simulink model "sf_frame_sync_controller"  (R2017b)
settings: Solver=FixedStepDiscrete  StartTime=0.0  StopTime=10.0  FixedStep=0.05  RelTol=1e-3  EnableMultiTasking=on
model workspace (MAT data in the model file):
  trainSig = [-0.707106781187+0.707106781187i; -0.707106781187+0.707106781187i; -0.707106781187+0.707106781187i; -0.707106781187+0.707106781187i; -0.707106781187-0.707106781187i; -0.707106781187-0.707106781187i; 0.707106781187-0.707106781187i; 0.707106781187-0.707106781187i; -0.707106781187-0.707106781187i; -0.707106781187+0.707106781187i; 0.707106781187-0.707106781187i; -0.707106781187-0.707106781187i; -0.707106781187+0.707106781187i; 0.707106781187-0.707106781187i; 0.707106781187-0.707106781187i; -0.707106781187-0.707106781187i; -0.707106781187-0.707106781187i; -0.707106781187-0.707106781187i; 0.707106781187+0.707106781187i; -0.707106781187+0.707106781187i; -0.707106781187+0.707106781187i; 0.707106781187+0.707106781187i; 0.707106781187-0.707106781187i; 0.707106781187+0.707106781187i; 0.707106781187+0.707106781187i; 0.707106781187+0.707106781187i; 0.707106781187+0.707106781187i; -0.707106781187+0.707106781187i; -0.707106781187+0.707106781187i; 0.707106781187-0.707106781187i; -0.707106781187+0.707106781187i; 0.707106781187+0.707106781187i; 0.707106781187-0.707106781187i; 0.707106781187-0.707106781187i; -0.707106781187+0.707106781187i; 0.707106781187+0.707106781187i; -0.707106781187+0.707106781187i; -0.707106781187+0.707106781187i; -0.707106781187-0.707106781187i; -0.707106781187+0.707106781187i; -0.707106781187-0.707106781187i; -0.707106781187-0.707106781187i; 0.707106781187+0.707106781187i; 0.707106781187+0.707106781187i; -0.707106781187+0.707106781187i; -0.707106781187+0.707106781187i; -0.707106781187+0.707106781187i; -0.707106781187-0.707106781187i; 0.707106781187+0.707106781187i; -0.707106781187+0.707106781187i; 0.707106781187-0.707106781187i; 0.707106781187+0.707106781187i; 0.707106781187-0.707106781187i; -0.707106781187-0.707106781187i; -0.707106781187+0.707106781187i; -0.707106781187-0.707106781187i; 0.707106781187+0.707106781187i; -0.707106781187+0.707106781187i; 0.707106781187-0.707106781187i; -0.707106781187-0.707106781187i; -0.707106781187-0.707106781187i; 0.707106781187+0.707106781187i; -0.707106781187+0.707106781187i; -0.707106781187-0.707106781187i]
settings Model: Creator=The MathWorks, Inc.  LastModifiedBy=The MathWorks, Inc.
settings DataIOCC: LimitDataPoints=on  SaveFormat=StructureWithTime  SaveOutput=off  SignalLogging=off  SaveTime=off
settings OptimizationCC: ExpressionDepthLimit=2147483647  InitFltsAndDblsToZero=on  EfficientMapNaN2IntZero=off  LifeSpan=inf
settings DebuggingCC: UnderspecifiedInitializationDetection=Classic  MergeDetectMultiDrivingBlocksExec=none  FcnCallInpInsideContextMsg=warning  StateNameClashWarn=warning  StrictBusMsg=Warning  SFUnexpectedBacktrackingDiag=warning  SFNoUnconditionalDefaultTransitionDiag=warning  SFExecutionAtInitializationDiag=none
settings HardwareCC: ProdBitPerPointer=32  ProdBitPerSizeT=32  ProdBitPerPtrDiffT=32  ProdLargestAtomicFloat=None  ProdIntDivRoundTo=Undefined  ProdEndianess=Unspecified  ProdWordSize=32  ProdHWDeviceType=32-bit Generic
settings ModelReferenceCC: PropagateSignalLabelsOutOfModel=off
settings SFSimCC: SimParseCustomCode=off
settings CodeAppCC: StateflowObjectComments=on
settings GRTTargetCC: TargetLangStandard=C89/C90 (ANSI)  GeneratePreprocessorConditionals=Disable all  CombineOutputUpdateFcns=off  GRTInterface=on
settings ConfigComp: CovMetricSettings=dw  CovHtmlReporting=on  CovSaveCumulativeToWorkspaceVar=on  CovSaveSingleToWorkspaceVar=on  CovExternalEMLEnable=off  CovSFcnEnable=off

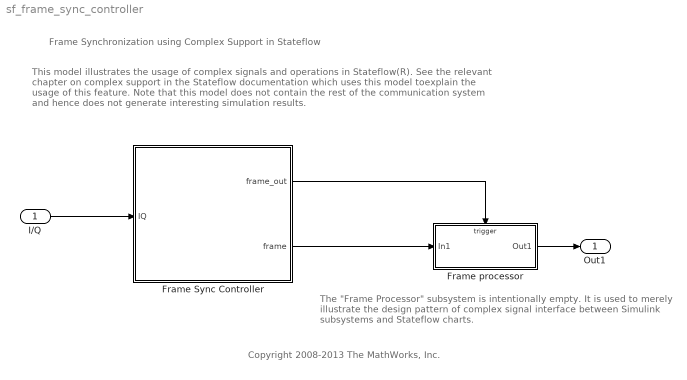
== system sf_frame_sync_controller ==
  note: This model illustrates the usage of complex signals and operations in Stateflow(R).
      | See the relevant chapter on complex support in the Stateflow documentation which uses
      | this model toexplain the usage of this feature. Note that this model does not contain the
      | rest of the communication system and hence does not generate interesting simulation results.
  note: Frame Synchronization using Complex Support in Stateflow
  note: The "Frame Processor" subsystem is intentionally empty.
      | It is used to merely illustrate the design pattern of complex signal interface
      | between Simulink subsystems and Stateflow charts.
  note: Copyright 2008-2013 The MathWorks, Inc.
  I/Q : Inport
  Frame Sync Controller : Stateflow chart  TreatAsAtomicUnit=on
  Frame processor : Subsystem  TreatAsAtomicUnit=on
  Out1 : Outport
  wires:
  I/Q/1 -> Frame Sync Controller/1(IQ)
  Frame Sync Controller/2(frame) -> Frame processor/1(In1)
  Frame Sync Controller/1(" frame_out") -> Frame processor/Trigger
  Frame processor/1(Out1) -> Out1/1

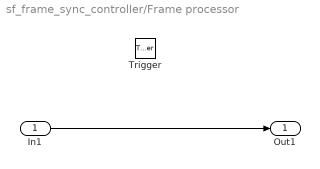
== system sf_frame_sync_controller/Frame processor ==
  In1 : Inport
  Trigger : TriggerPort  VariantControl=(inherit)
  Out1 : Outport
  wires:
  In1/1 -> Out1/1

== stateflow chart sf_frame_sync_controller/Frame Sync Controller ==
  state look_for_sync
    en:
    corrAbs = 0;
    du:
    [corr, corrAbs] = correlate(IQ);
  state frame_out
  state get_payload
    en:
    phasor = get_carrier_phase(corr);
    frame[0] = IQ * phasor;
    du:
    frame[temporalCount(tick)] = IQ * phasor;
  (default) -> look_for_sync
  frame_out -> look_for_sync
  look_for_sync -> frame_out [order 2] : [after(300,tick)]
      | {frame = 0;}
  look_for_sync -> get_payload [order 1] : [corrAbs > 50]
  get_payload -> frame_out : [after(220,tick)]
  data: u function_input double; y function_output double; yabs function_output double; u function_input double; y function_output double; IQ input double; phasor local double; corr local double; corrAbs local double; frame_out output boolean; frame output double size=221; trainSig local double size=64
  function [y, yabs] = correlate(u):
    | function [y, yabs] = correlate(u)
    | 
    | persistent zi;
    | 
    | B = conj(flipud(trainSig));
    | A = 1;
    | 
    | if(isempty(zi))
    |     zi = zeros(max(length(A),length(B))-1,1) + complex(0,0);
    | end
    | 
    | [y,zi] = filter(B,A,u,zi);
    | 
    | yabs = abs(y);
  function y = get_carrier_phase(u):
    | function y = get_carrier_phase(u)
    | 
    | y = exp(-1i*angle(u));
